simulink model "DebuggingModel_1"  (R2022b)
settings: Solver=VariableStepAuto  StartTime=0.0  StopTime=10.0  RelTol=1e-3
model workspace (MAT data in the model file):
  accumulated_data = 0
libraries: VACLib x3
settings Model: Creator=KarlO  LastModifiedBy=JMESSING

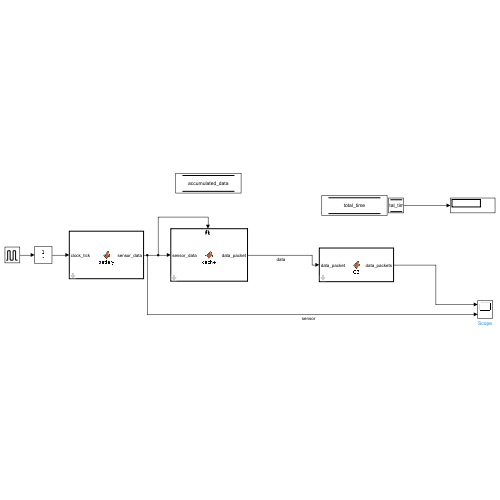
[thumbnail: Simulink's stored preview of the top-level diagram]
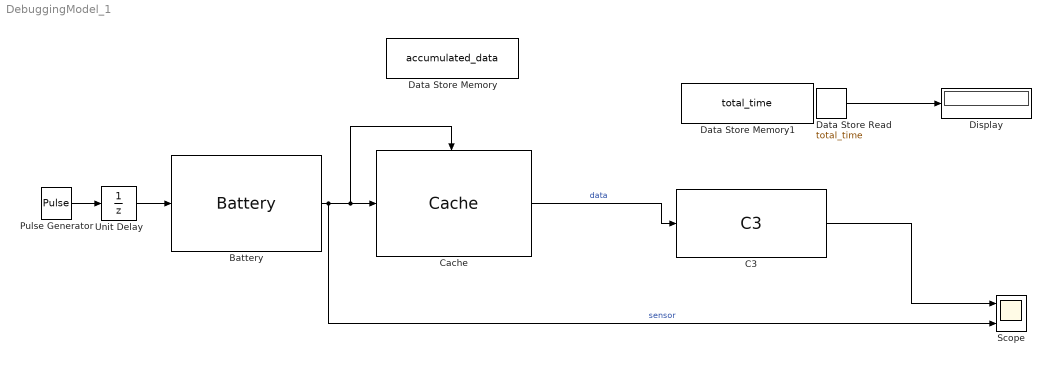
== system DebuggingModel_1 ==
  Battery : VACLib/Sources/Battery  sensor_data_size=8
      settings: LibrarySourceBlock=|
      | simulink/User-Defined
      | Functions/MATLAB Function
  C3 : VACLib/AWS Components/C3  mask{consistency=0, total_time=0}
      mask prompts: total_time "Total Time"
      settings: LibrarySourceBlock=|
      | simulink/User-Defined
      | Functions/MATLAB Function
  Cache : VACLib/Vehicle Components/Cache  cache_size=32
      settings: LibrarySourceBlock=|
      | simulink/User-Defined
      | Functions/MATLAB Function
  Data Store Memory : DataStoreMemory  DataStoreName=accumulated_data  WriteAfterWriteMsg=warning  ShowAdditionalParam=off  OutDataTypeStr=double
  Data Store Memory1 : DataStoreMemory  DataStoreName=total_time  WriteAfterWriteMsg=warning  ShowAdditionalParam=off  OutDataTypeStr=double
  Data Store Read : DataStoreRead  DataStoreName=total_time  IndexOptions=Index vector (dialog)  Indices=1  OutputSizes=1
  Display : Display
  Pulse Generator : DiscretePulseGenerator  PulseType=Time based  PulseWidth=50
  Scope : Scope  NumInputPorts=2
  Unit Delay : UnitDelay  SampleTime=-1  HasFrameUpgradeWarning=on
  wires:
  Cache/1 -> C3/1  "data"
  Battery/1 -> Cache/Trigger, Cache/1, Scope/2  "sensor"
  Pulse Generator/1 -> Unit Delay/1
  Unit Delay/1 -> Battery/1
  C3/1 -> Scope/1
  Data Store Read/1 -> Display/1
